simulink model "WDS_evaluate_detector"  (R2022a)
settings: Solver=FixedStepDiscrete  StartTime=0.0  StopTime=T_final  FixedStep=T_sample  RelTol=1e-3
values from neighbouring files (symbols this model uses):
  A_bar_d = readmatrix('A_bar_d.csv')    [Run_model_WDS.m]
  B_bar_d = readmatrix('B_bar_d.csv')    [Run_model_WDS.m]
  BDD_thresh = 5    [Run_model_WDS.m]    (also in run_model.m = 0.05)
  C_obsv_d = readmatrix('C_obsv_d.csv')    [Run_model_WDS.m]    (also in run_model.m = C_obsv; run_model_power_system.m = C_obsv)
  Cm = ones(1,n_states)    [Run_model_WDS.m]
  D_obsv_d = readmatrix('D_obsv_d.csv')    [Run_model_WDS.m]    (also in run_model.m = D_obsv; run_model_power_system.m = D_obsv)
  K = place(A_bar_d,B_bar_d,Pc)    [Run_model_WDS.m]
  max_attack = 1000    [Run_model_WDS.m]
  n_attack = round(attack_percentage*n_meas)    [Run_model_WDS.m]    (also in run_model.m = round(0.2*n_meas))
  n_meas = size(C_obsv_d,1)    [Run_model_WDS.m]    (also in run_model.m = n_gen + n_bus; run_model_power_system.m = n_gen + n_bus)
  offset = -inv(B_bar_d)*(A_bar_d-eye(n_states))*xd    [Run_model_WDS.m]
  r_tau = chi2inv(0.1,n_meas)    [Run_model_WDS.m]
  Sigma = diag(sigma)    [Run_model_WDS.m]    (also in run_model.m)
  sigma_inv_k = 1e2*(3 + 2*rand(n_meas,1))    [Run_model_WDS.m]    (also in run_model.m = 1e4*(3 + 2*rand(m,1)); sigma_inv_k.mat = [541957.05841 17086.3156535 20847.4062112 958.936090052 8825)
  T_sample = 0.01    [Run_model_WDS.m]    (also in run_model.m; run_model_power_system.m)
  T_start_attack = 0.1*T_final    (= 0.8)    [Run_model_WDS.m]    (also in run_model.m = 1.6; run_model_power_system.m)
  x0 = zeros(n_states,1)    [Run_model_WDS.m]    (also in run_model.m; run_model_power_system.m)
  xd = 5*ones(n_states,1)    [Run_model_WDS.m]
libraries: simulink x2
settings Model: Creator=Abelb  LastModifiedBy=Abelb

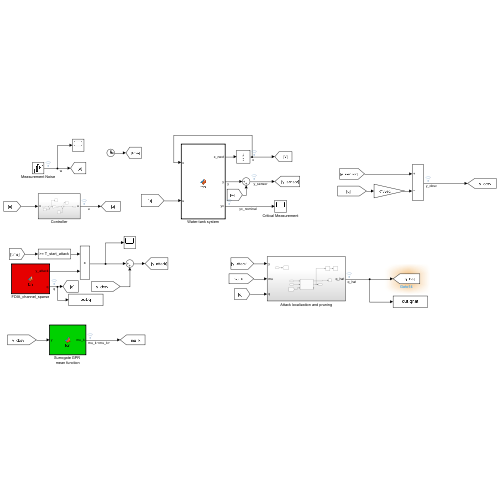
[thumbnail: Simulink's stored preview of the top-level diagram]
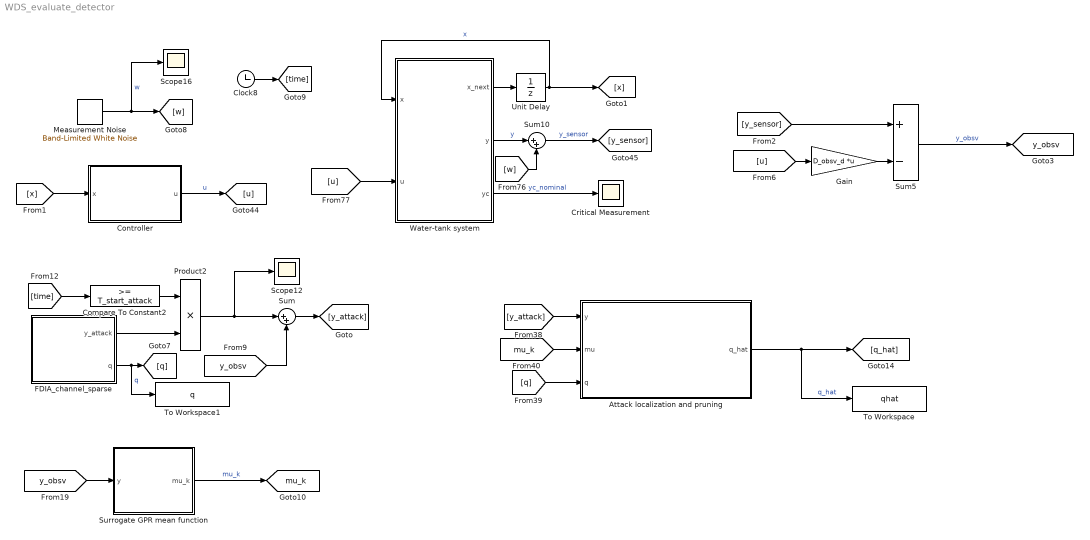
== system WDS_evaluate_detector ==
  Attack localization and pruning : Subsystem
  Clock8 : Clock
  Compare To Constant2 : simulink/Logic and Bit Operations/Compare To Constant  relop=>=  const=T_start_attack  OutDataTypeStr=boolean
  Controller : Subsystem
  Critical Measurement : Scope
  FDIA_channel_sparse : MATLAB Function  TreatAsAtomicUnit=on
  Gain : Gain  Gain=D_obsv_d  Multiplication=Matrix(K*u) (u vector)
  Measurement Noise : simulink/Sources/Band-Limited White Noise  Cov=[1e-7]  Ts=T_sample  seed=[23341]
  Product2 : Product
  Scope12 : Scope
  Scope16 : Scope
  Sum : Sum  Inputs=|++
  Sum10 : Sum  Inputs=|++
  Sum5 : Sum  Inputs=+-
  Surrogate GPR mean function : MATLAB Function  TreatAsAtomicUnit=on
  To Workspace : ToWorkspace  VariableName=qhat  SaveFormat=Timeseries  SampleTime=-1
  To Workspace1 : ToWorkspace  VariableName=q  SaveFormat=Timeseries  SampleTime=-1
  Unit Delay : UnitDelay  InitialCondition=x0  SampleTime=-1  HasFrameUpgradeWarning=on
  Water-tank system : MATLAB Function  TreatAsAtomicUnit=on
  tag scope: mu_k=global, y_obsv=global
  wires:
  Measurement Noise/1 -> Scope16/1, [w]  "w"
  Unit Delay/1 -> Water-tank system/1(x), [x]  "x"
  Water-tank system/3(yc) -> Critical Measurement/1  "yc_nominal"
  [w] -> Sum10/2
  [x] -> Controller/1(x)
  [u] -> Water-tank system/2(u)
  Sum10/1 -> [y_sensor]  "y_sensor"
  Controller/1(u) -> [u]  "u"
  Water-tank system/2(y) -> Sum10/1  "y"
  Water-tank system/1(x_next) -> Unit Delay/1
  [y_sensor] -> Sum5/1
  [u] -> Gain/1
  Gain/1 -> Sum5/2
  Sum5/1 -> [y_obsv]  "y_obsv"
  FDIA_channel_sparse/1(y_attack) -> Product2/2
  FDIA_channel_sparse/2(q) -> To Workspace1/1, [q]  "q"
  [time] -> Compare To Constant2/1
  Compare To Constant2/1 -> Product2/1
  Product2/1 -> Scope12/1, Sum/1
  [y_obsv] -> Sum/2
  Sum/1 -> [y_attack]
  [y_obsv] -> Surrogate GPR mean function/1(y)
  Surrogate GPR mean function/1(mu_k) -> [mu_k]  "mu_k"
  Clock8/1 -> [time]
  [mu_k] -> Attack localization and pruning/2(mu)
  [y_attack] -> Attack localization and pruning/1(y)
  [q] -> Attack localization and pruning/3(q)
  Attack localization and pruning/1(q_hat) -> To Workspace/1, [q_hat]  "q_hat"

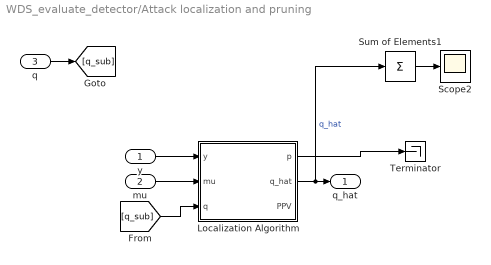
== system WDS_evaluate_detector/Attack localization and pruning ==
  y : Inport
  mu : Inport  Port=2
  q : Inport  Port=3
  Localization Algorithm : MATLAB Function  TreatAsAtomicUnit=on
  Scope2 : Scope
  Sum of Elements1 : Sum  Inputs=+
  Terminator : Terminator
  q_hat : Outport
  wires:
  y/1 -> Localization Algorithm/1(y)
  mu/1 -> Localization Algorithm/2(mu)
  Localization Algorithm/2(q_hat) -> Sum of Elements1/1, q_hat/1  "q_hat"
  q/1 -> [q_sub]
  [q_sub] -> Localization Algorithm/3(q)
  Sum of Elements1/1 -> Scope2/1
  Localization Algorithm/1(p) -> Terminator/1

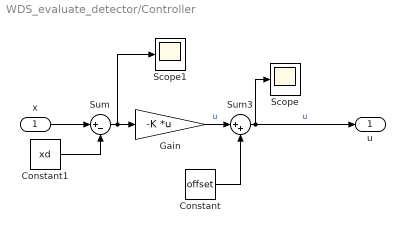
== system WDS_evaluate_detector/Controller ==
  x : Inport
  Constant : Constant  Value=offset
  Constant1 : Constant  Value=xd
  Gain : Gain  Gain=-K  Multiplication=Matrix(K*u) (u vector)
  Scope : Scope
  Scope1 : Scope
  Sum : Sum  Inputs=|+-
  Sum3 : Sum  Inputs=|++
  u : Outport
  wires:
  Sum3/1 -> u/1, Scope/1  "u"
  Constant/1 -> Sum3/2
  Constant1/1 -> Sum/2
  Gain/1 -> Sum3/1  "u"
  Sum/1 -> Scope1/1, Gain/1
  x/1 -> Sum/1

== matlab function WDS_evaluate_detector/Surrogate GPR mean function ==
  data: y input; mu_k output; sigma_inv_k parameter; r_tau parameter; n_meas parameter
function mu_k = fcn(y,sigma_inv_k, r_tau,n_meas)
% Prunes a random vector to find mu_k so that ||y-mu_k||_Sigma_inv_k <= r_tau

% first: random vector, secomd: normalize
y_rand = rand(n_meas,1);
y_rand = sqrt(r_tau/max(sigma_inv_k))/norm(y_rand)*y_rand;

% create mu_k from y
mu_k = y - y_rand;

% mu_k = (U_y_1*U_y_1.')*y;

== matlab function WDS_evaluate_detector/FDIA_channel_sparse ==
  data: n_attack parameter; y_attack output; n_meas parameter; C_obsv_d parameter; max_attack parameter; BDD_thresh parameter; q output
function [y_attack,q] = fcn(n_attack,n_meas,C_obsv_d,max_attack, BDD_thresh)

%% Measurement Channel Attack
%  Assumptions:
%  1. The attacker knows the actual measurement
%  2. The attacker can only corrupt upto n_attack measurements
%  3. The attacker knows the BDD theshold

attack_idx = randi(n_meas,n_attack,1);
% attack_idx = [10; 18];
y_attack   = gen_attack_channel(C_obsv_d, max_attack,attack_idx,BDD_thresh);
                                                        % NOTE THE .75
                                                        % Used
                                                        % conservatively
q = ones(n_meas,1);
q(attack_idx) = 0;

== matlab function WDS_evaluate_detector/Attack localization and pruning/Localization Algorithm ==
  data: p output; y input; q_hat output; mu input; Sigma parameter; n_meas parameter; q input; PPV output
function [p, q_hat,PPV] = fcn(y,mu,Sigma, n_meas,q)

%% calculate probability
z = (y - mu)./diag(Sigma);
p = 2*(ones(n_meas,1)-normcdf(abs(z)));

%% support prior and corresponding confidence
% q_hat = zeros(n_meas,1);
% q_hat(p <= 0.5) = 1;
q_hat = double(p>=0.5);

PPV = sum(q.*q_hat)/sum(q_hat);

== matlab function WDS_evaluate_detector/Water-tank system ==
  data: x input; x_next output; u input; y output; A_bar_d parameter; C_obsv_d parameter; B_bar_d parameter; D_obsv_d parameter; yc output; Cm parameter
function [x_next,y,yc] = fcn(x,u,A_bar_d,C_obsv_d,B_bar_d,D_obsv_d,Cm)
% Discrete state-space model for system

x_next = A_bar_d*x + B_bar_d*u ;

y = C_obsv_d*x + D_obsv_d*u;

% critical measurements
yc = Cm*x;
